simulink model "ebike"  (Simulink 8.1)
settings: Solver=ode3  StartTime=0.0  StopTime=0.3  FixedStep=0.001  MaxStep=0.001  MinStep=0.001  RelTol=1e-3
values from neighbouring files (symbols this model uses):
  A = 0.38    [run_sim.m]
  Cr = 0.003    [run_sim.m]
  Cw = 0.4    [run_sim.m]
libraries: simulink x2
settings Model: Creator=stwei  LastModifiedBy=Shahabaz
settings DataIOCC: SignalLoggingSaveFormat=Dataset  SaveOutput=off  SignalLogging=off
settings GRTTargetCC: CodeReplacementLibrary=None  CPPClassGenCompliant=on

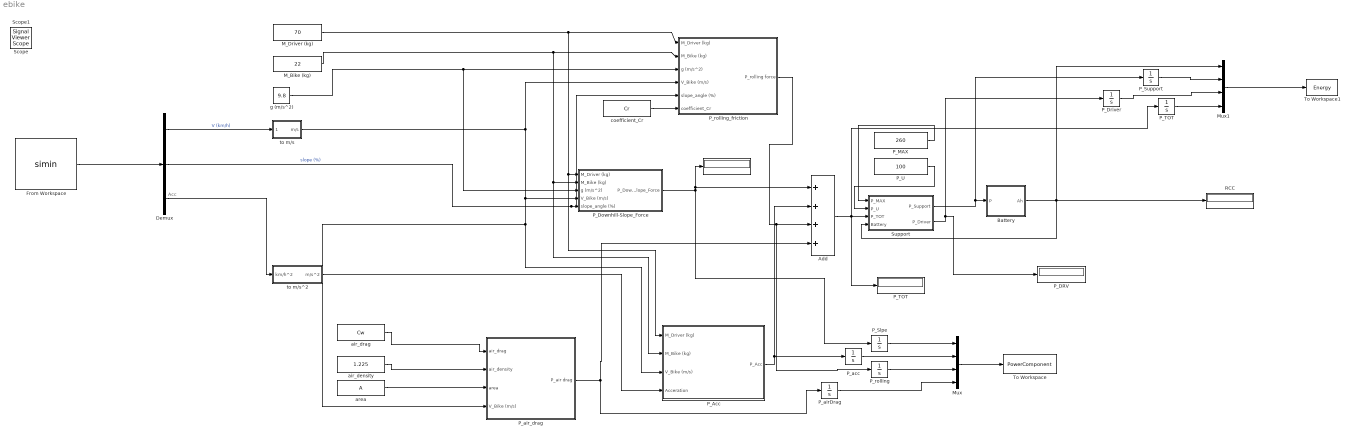
== system ebike ==
  note: Acc
  "   " : Display
  " P_DRV" : Display
  " P_TOT" : Display
  Add : Sum  Inputs=++++
  Battery : Subsystem
  Demux : Demux  Outputs=3
  From Workspace : FromWorkspace  VariableName=simin  SampleTime=0  OutputAfterFinalValue=Setting to zero
  M_Bike (kg) : Constant  Value=22
  M_Driver (kg) : Constant  Value=70
  Mux : Mux
  Mux1 : Mux
  P_Acc : Subsystem
  P_Downhill-Slope_Force : Subsystem
  "P_Driver " : Integrator
  P_MAX : Constant  Value=260
  P_Slpe : Integrator
  P_Support : Integrator
  P_TOT : Integrator
  P_U : Constant  Value=100
  P_acc : Integrator
  P_airDrag : Integrator
  "P_air_drag " : Subsystem
  P_rolling : Integrator
  "P_rolling_friction " : Subsystem
  RCC : Display
  Support : Subsystem
  To Workspace : ToWorkspace  VariableName=PowerComponent
  To Workspace1 : ToWorkspace  VariableName=Energy
  air_density : Constant  Value=1.225
  air_drag : Constant  Value=Cw
  area : Constant  Value=A
  coefficient_Cr : Constant  Value=Cr
  g (m/s^2) : Constant  Value=9.8
  to m/s : Subsystem
  to m/s^2 : Subsystem
  Scope : SignalViewerScope  IOType=viewer  RefreshTime=0.035000
  Scope1 : SignalViewerScope  IOType=viewer  RefreshTime=0.035000
  wires:
  M_Driver (kg)/1 -> P_Acc/1(M_Driver (kg)), P_Downhill-Slope_Force/1(M_Driver (kg)), "P_rolling_friction "/1(M_Driver (kg))
  M_Bike (kg)/1 -> P_Acc/2(M_Bike (kg)), P_Downhill-Slope_Force/2(M_Bike (kg)), "P_rolling_friction "/2(M_Bike (kg))
  g (m/s^2)/1 -> P_Downhill-Slope_Force/3(g (m/s^2)), "P_rolling_friction "/3(g (m/s^2))
  to m/s/1(m/s) -> "P_rolling_friction "/4(V_Bike (m/s)), P_Acc/3(V_Bike (m/s)), "P_air_drag "/4(V_Bike (m/s)), P_Downhill-Slope_Force/4(V_Bike (m/s))
  P_MAX/1 -> Support/1(P_MAX)
  P_U/1 -> Support/2(P_U)
  Support/1(P_Support) -> P_Support/1, Battery/1(P)
  Support/2(P_Driver) -> "P_Driver "/1, " P_DRV"/1
  Battery/1(Ah) -> Mux1/1, RCC/1, Support/4(Battery)
  From Workspace/1 -> Demux/1
  Demux/1 -> to m/s/1(km/h)  "V (km/h)"
  Demux/2 -> "P_rolling_friction "/5(slope_angle (%)), P_Downhill-Slope_Force/5(slope_angle (%))  "slope (%)"
  to m/s^2/1(m/s^2) -> P_Acc/4("Acceration ")
  air_drag/1 -> "P_air_drag "/1(air_drag)
  air_density/1 -> "P_air_drag "/2(air_density)
  area/1 -> "P_air_drag "/3(area)
  coefficient_Cr/1 -> "P_rolling_friction "/6(coefficient_Cr)
  Demux/3 -> to m/s^2/1(km/h^2)
  Mux/1 -> To Workspace/1
  Mux1/1 -> To Workspace1/1
  "P_rolling_friction "/1(P_rolling force) -> P_rolling/1, Add/3
  "P_air_drag "/1(P_air drag) -> Add/4, P_airDrag/1
  P_Support/1 -> Mux1/2
  "P_Driver "/1 -> Mux1/3
  P_TOT/1 -> Mux1/4
  P_Downhill-Slope_Force/1(P_Downhill-Slope_Force) -> "   "/1, Add/1, P_Slpe/1
  P_Acc/1(P_Acc) -> Add/2, P_acc/1
  P_rolling/1 -> Mux/3
  P_airDrag/1 -> Mux/4
  P_acc/1 -> Mux/2
  P_Slpe/1 -> Mux/1
  Add/1 -> P_TOT/1, " P_TOT"/1, Support/3(P_TOT)

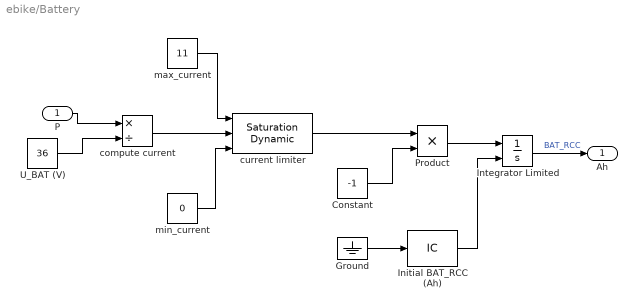
== system ebike/Battery ==
  P : Inport
  Constant : Constant  Value=-1
  Ground : Ground
  Initial BAT_RCC (Ah) : InitialCondition  Value=11
  Integrator Limited : Integrator  InitialConditionSource=external  LimitOutput=on  UpperSaturationLimit=13  LowerSaturationLimit=0
  Product : Product  RndMeth=Zero
  U_BAT (V) : Constant  Value=36
  compute current : Product  Inputs=*/
  current limiter : simulink/Discontinuities/Saturation Dynamic  OutMin=[]  OutMax=[]  OutDataTypeStr=Inherit: Same as second input  OutDataType=fixdt(1, 16)  OutScaling=2^-10  DoSatur=on
  max_current : Constant  Value=11
  min_current : Constant  Value=0
  Ah : Outport
  wires:
  Ground/1 -> Initial BAT_RCC (Ah)/1
  U_BAT (V)/1 -> compute current/2
  Initial BAT_RCC (Ah)/1 -> Integrator Limited/2
  Constant/1 -> Product/2
  Product/1 -> Integrator Limited/1
  P/1 -> compute current/1
  Integrator Limited/1 -> Ah/1  "BAT_RCC"
  current limiter/1 -> Product/1
  compute current/1 -> current limiter/2
  max_current/1 -> current limiter/1
  min_current/1 -> current limiter/3

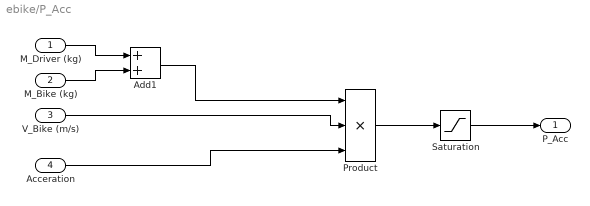
== system ebike/P_Acc ==
  M_Driver (kg) : Inport
  M_Bike (kg) : Inport  Port=2
  V_Bike (m/s) : Inport  Port=3
  "Acceration " : Inport  Port=4
  Add1 : Sum
  Product : Product  Inputs=3  RndMeth=Zero
  Saturation : Saturate  UpperLimit=10000  LowerLimit=0
  P_Acc : Outport
  wires:
  Add1/1 -> Product/1
  M_Driver (kg)/1 -> Add1/1
  M_Bike (kg)/1 -> Add1/2
  V_Bike (m/s)/1 -> Product/2
  Product/1 -> Saturation/1
  Saturation/1 -> P_Acc/1
  "Acceration "/1 -> Product/3

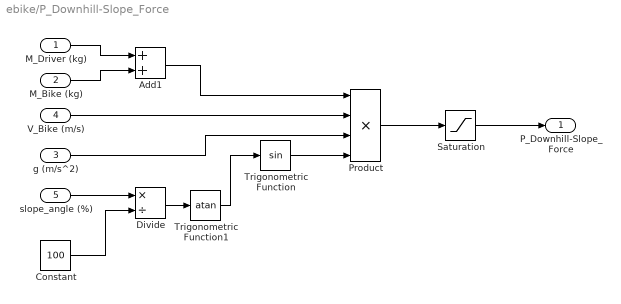
== system ebike/P_Downhill-Slope_Force ==
  M_Driver (kg) : Inport
  M_Bike (kg) : Inport  Port=2
  g (m/s^2) : Inport  Port=3
  V_Bike (m/s) : Inport  Port=4
  slope_angle (%) : Inport  Port=5
  Add1 : Sum
  Constant : Constant  Value=100
  Divide : Product  Inputs=*/
  Product : Product  Inputs=4  RndMeth=Zero
  Saturation : Saturate  UpperLimit=10000  LowerLimit=0
  Trigonometric Function : Trigonometry
  Trigonometric Function1 : Trigonometry  Operator=atan
  P_Downhill-Slope_Force : Outport
  wires:
  Add1/1 -> Product/1
  M_Driver (kg)/1 -> Add1/1
  M_Bike (kg)/1 -> Add1/2
  V_Bike (m/s)/1 -> Product/2
  g (m/s^2)/1 -> Product/3
  Trigonometric Function/1 -> Product/4
  Trigonometric Function1/1 -> Trigonometric Function/1
  slope_angle (%)/1 -> Divide/1
  Divide/1 -> Trigonometric Function1/1
  Constant/1 -> Divide/2
  Product/1 -> Saturation/1
  Saturation/1 -> P_Downhill-Slope_Force/1

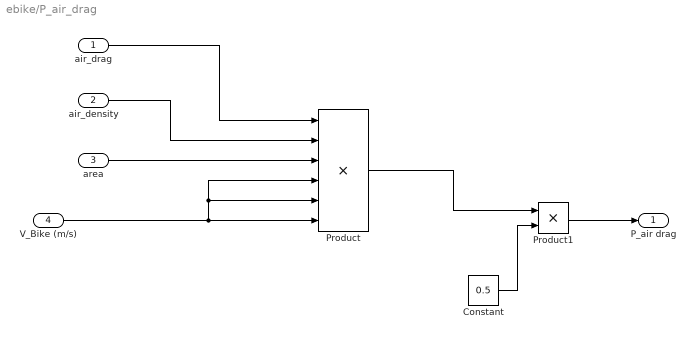
== system ebike/P_air_drag  ==
  air_drag : Inport
  air_density : Inport  Port=2
  area : Inport  Port=3
  V_Bike (m/s) : Inport  Port=4
  Constant : Constant  Value=0.5
  Product : Product  Inputs=6  RndMeth=Zero
  Product1 : Product
  P_air drag : Outport
  wires:
  air_drag/1 -> Product/1
  air_density/1 -> Product/2
  area/1 -> Product/3
  Product/1 -> Product1/1
  Constant/1 -> Product1/2
  Product1/1 -> P_air drag/1
  V_Bike (m/s)/1 -> Product/6, Product/5, Product/4

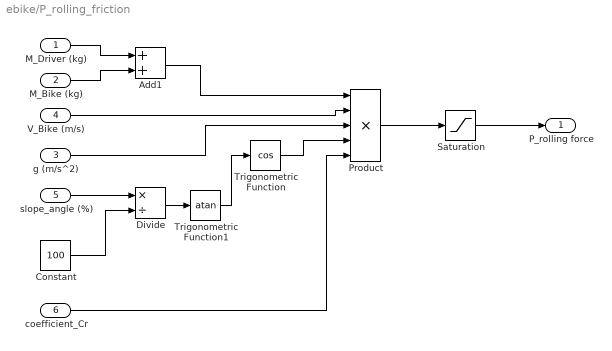
== system ebike/P_rolling_friction  ==
  M_Driver (kg) : Inport
  M_Bike (kg) : Inport  Port=2
  g (m/s^2) : Inport  Port=3
  V_Bike (m/s) : Inport  Port=4
  slope_angle (%) : Inport  Port=5
  coefficient_Cr : Inport  Port=6
  Add1 : Sum
  Constant : Constant  Value=100
  Divide : Product  Inputs=*/
  Product : Product  Inputs=5  RndMeth=Zero
  Saturation : Saturate  UpperLimit=10000  LowerLimit=0
  Trigonometric Function : Trigonometry  Operator=cos
  Trigonometric Function1 : Trigonometry  Operator=atan
  P_rolling force : Outport
  wires:
  Add1/1 -> Product/1
  M_Driver (kg)/1 -> Add1/1
  M_Bike (kg)/1 -> Add1/2
  V_Bike (m/s)/1 -> Product/2
  g (m/s^2)/1 -> Product/3
  Trigonometric Function/1 -> Product/4
  Trigonometric Function1/1 -> Trigonometric Function/1
  slope_angle (%)/1 -> Divide/1
  Divide/1 -> Trigonometric Function1/1
  Constant/1 -> Divide/2
  Product/1 -> Saturation/1
  Saturation/1 -> P_rolling force/1
  coefficient_Cr/1 -> Product/5

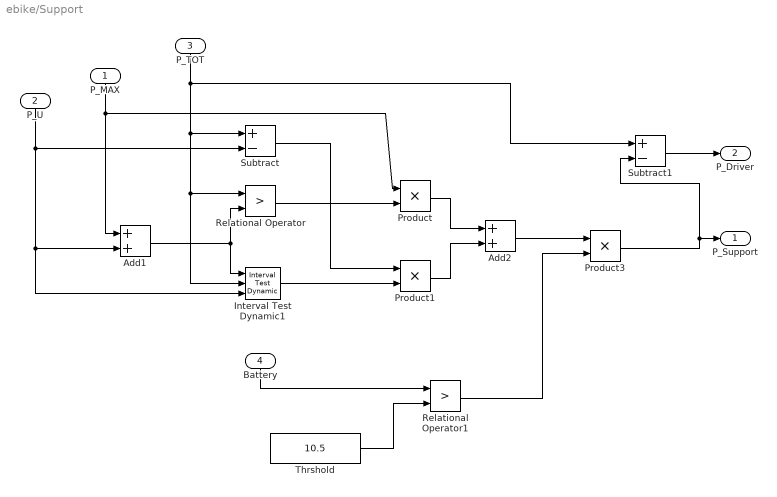
== system ebike/Support ==
  P_MAX : Inport
  P_U : Inport  Port=2
  P_TOT : Inport  Port=3
  Battery : Inport  Port=4
  Add1 : Sum
  Add2 : Sum
  Interval Test Dynamic1 : simulink/Logic and Bit Operations/Interval Test Dynamic  IntervalClosedRight=on  IntervalClosedLeft=on  OutDataTypeStr=uint8
  Product : Product  RndMeth=Zero
  Product1 : Product  RndMeth=Zero
  Product3 : Product  RndMeth=Zero
  Relational Operator : RelationalOperator  Operator=>  OutDataTypeStr=boolean
  Relational Operator1 : RelationalOperator  Operator=>  OutDataTypeStr=boolean
  Subtract : Sum  Inputs=+-
  Subtract1 : Sum  Inputs=+-
  Thrshold : Constant  Value=10.5
  P_Support : Outport
  P_Driver : Outport  Port=2
  wires:
  Add1/1 -> Interval Test Dynamic1/1, Relational Operator/2
  P_TOT/1 -> Subtract1/1, Subtract/1, Interval Test Dynamic1/2, Relational Operator/1
  P_U/1 -> Subtract/2, Interval Test Dynamic1/3, Add1/2
  P_MAX/1 -> Product/1, Add1/1
  Relational Operator/1 -> Product/2
  Subtract/1 -> Product1/1
  Interval Test Dynamic1/1 -> Product1/2
  Product/1 -> Add2/1
  Product1/1 -> Add2/2
  Add2/1 -> Product3/1
  Subtract1/1 -> P_Driver/1
  Relational Operator1/1 -> Product3/2
  Battery/1 -> Relational Operator1/1
  Product3/1 -> P_Support/1, Subtract1/2
  Thrshold/1 -> Relational Operator1/2

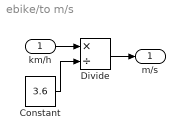
== system ebike/to m/s ==
  km/h : Inport
  Constant : Constant  Value=3.6
  Divide : Product  Inputs=*/
  m/s : Outport
  wires:
  Constant/1 -> Divide/2
  km/h/1 -> Divide/1
  Divide/1 -> m/s/1

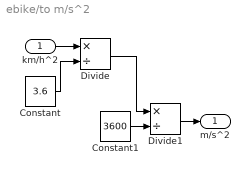
== system ebike/to m/s^2 ==
  km/h^2 : Inport
  Constant : Constant  Value=3.6
  Constant1 : Constant  Value=3600
  Divide : Product  Inputs=*/
  Divide1 : Product  Inputs=*/
  m/s^2 : Outport
  wires:
  Constant/1 -> Divide/2
  km/h^2/1 -> Divide/1
  Divide/1 -> Divide1/1
  Divide1/1 -> m/s^2/1
  Constant1/1 -> Divide1/2
